simulink model "cic_1000"  (Simulink 7.8)
settings: Solver=ode45  StartTime=0.0  StopTime=10.0  RelTol=1e-3
libraries: dspsigops x8, dspsrcs4 x1
settings Model: Creator=svenhoffmann  LastModifiedBy=josef  ExtModeAutoUpdateStatusClock=off
settings OptimizationCC: InitFltsAndDblsToZero=on
settings DebuggingCC: SaveWithParameterizedLinksMsg=none  SignalResolutionControl=TryResolveAllWithWarning  MultiTaskDSMMsg=warning  MultiTaskCondExecSysMsg=none  FcnCallInpInsideContextMsg=Use local settings  StrictBusMsg=None
settings RTWCC: IncludeERTFirstTime=on
settings GRTTargetCC: TargetFcnLib=ansi_tfl_tmw.mat

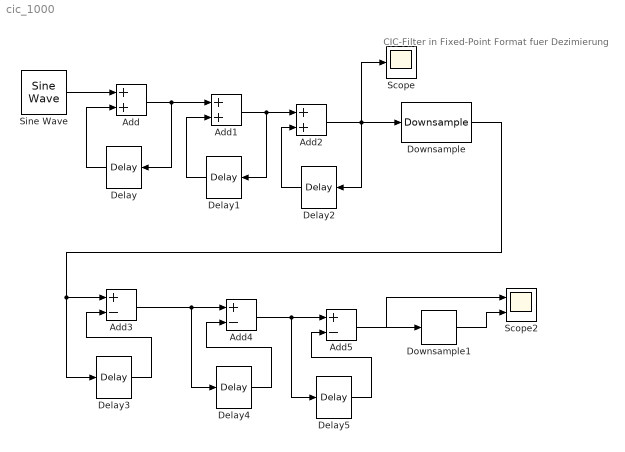
== system cic_1000 ==
  note: CIC-Filter
      | in Fixed-Point
      | Format
      | fuer Dezimierung
  Add : Sum  OutDataTypeStr=fixdt(1,38,0)
  Add1 : Sum  OutDataTypeStr=fixdt(1,38,0)
  Add2 : Sum  OutDataTypeStr=fixdt(1,38,0)
  Add3 : Sum  Inputs=+-
  Add4 : Sum  Inputs=+-
  Add5 : Sum  Inputs=+-
  Delay{,1..5} (6 alike) : dspsigops/Delay  dly_unit=Samples  delay=1  ic_detail=off  dif_ic_for_ch=off  dif_ic_for_dly=off  ic=0  reset_popup=None
  Downsample : dspsigops/Downsample  N=1000  phase=0  InputProcessing=Inherited (this choice will be removed - see release notes)  RateOptions=Enforce single-rate processing  smode=Allow multirate  fmode=Maintain input frame size  ic=0
  Downsample1 : dspsigops/Downsample  N=2  phase=0  InputProcessing=Inherited (this choice will be removed - see release notes)  RateOptions=Enforce single-rate processing  smode=Allow multirate  fmode=Maintain input frame size  ic=0
  Scope : Scope
  Scope2 : Scope  NumInputPorts=2
      settings: YMin=-1.25e+11~-1.25e+11  YMax=1.25e+11~1.25e+11  SaveName=ScopeData2
  Sine Wave : dspsrcs4/Sine Wave  Amplitude=127  Frequency=0.5  Phase=0  SampleMode=Discrete  OutComplex=Real  CompMethod=Table lookup  TableSize=Speed  SampleTime=1/10000  SamplesPerFrame=1  ResetState=Restart at time zero  dataType=Fixed-point  wordLen=38  udDataType=sfix(16)  fracBitsMode=User-defined  numFracBits=0  OutDataTypeStr=fixdt(1,38,0)  LastOutDataTypeStr=fixdt(1,38,0)
  wires:
  Sine Wave/1 -> Add/1
  Delay/1 -> Add/2
  Add/1 -> Add1/1, Delay/1
  Delay1/1 -> Add1/2
  Add1/1 -> Delay1/1, Add2/1
  Add2/1 -> Downsample/1, Scope/1, Delay2/1
  Delay2/1 -> Add2/2
  Delay3/1 -> Add3/2
  Delay4/1 -> Add4/2
  Delay5/1 -> Add5/2
  Add3/1 -> Delay4/1, Add4/1
  Add4/1 -> Delay5/1, Add5/1
  Downsample/1 -> Delay3/1, Add3/1
  Add5/1 -> Downsample1/1, Scope2/1
  Downsample1/1 -> Scope2/2
